simulink model "Simulacion_Variables_Estado"  (R2016a)
settings: Solver=VariableStepAuto  StartTime=0.0  StopTime=10.0  RelTol=1e-3
values from neighbouring files (symbols this model uses):
  b = [1;1]    [ejemplodiscretro.m]
undefined symbols (not defined in the file or in its folder): A, B, C, k, m
settings Model: Creator=Daniel  LastModifiedBy=Daniel

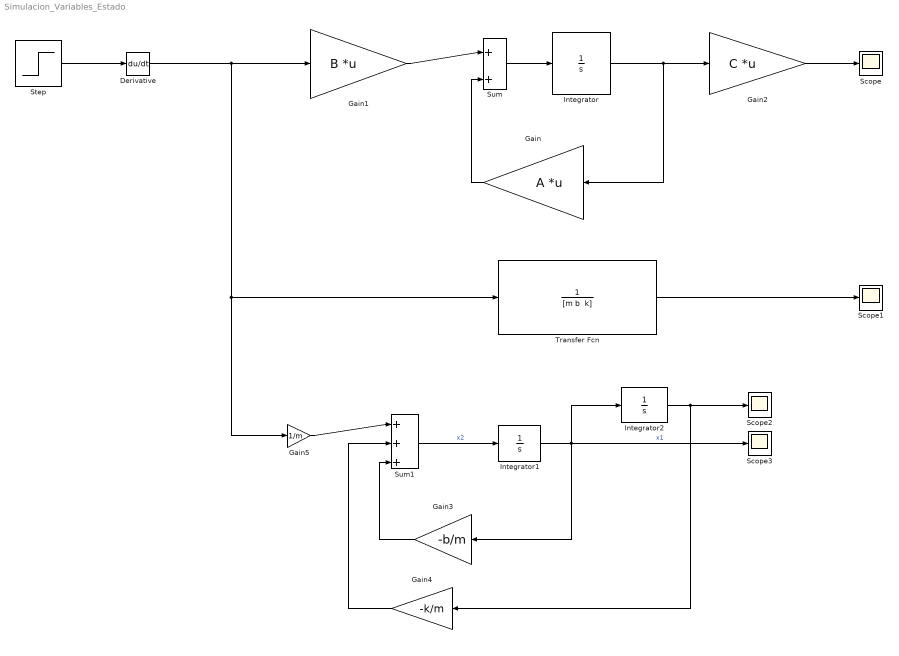
== system Simulacion_Variables_Estado ==
  Derivative : Derivative
  Gain : Gain  Gain=A  Multiplication=Matrix(K*u) (u vector)
  Gain1 : Gain  Gain=B  Multiplication=Matrix(K*u) (u vector)
  Gain2 : Gain  Gain=C  Multiplication=Matrix(K*u) (u vector)
  Gain3 : Gain  Gain=-b/m
  Gain4 : Gain  Gain=-k/m
  Gain5 : Gain  Gain=1/m
  Integrator : Integrator
  Integrator1 : Integrator
  Integrator2 : Integrator
  Scope{,1..3} (4 alike) : Scope
  Step : Step  SampleTime=0
  Sum : Sum  Inputs=|++
  Sum1 : Sum  Inputs=|+++
  Transfer Fcn : TransferFcn  Denominator="[m b  k]"
  wires:
  Gain1/1 -> Sum/1
  Sum/1 -> Integrator/1
  Integrator/1 -> Gain/1, Gain2/1
  Gain/1 -> Sum/2
  Gain2/1 -> Scope/1
  Step/1 -> Derivative/1
  Derivative/1 -> Transfer Fcn/1, Gain5/1, Gain1/1
  Transfer Fcn/1 -> Scope1/1
  Sum1/1 -> Integrator1/1  "x2"
  Integrator1/1 -> Scope3/1, Integrator2/1, Gain3/1  "x1"
  Gain3/1 -> Sum1/3
  Gain4/1 -> Sum1/2
  Gain5/1 -> Sum1/1
  Integrator2/1 -> Scope2/1, Gain4/1
